simulink model "Saturation"  (R2022b)
settings: Solver=VariableStepAuto  StartTime=0.0  StopTime=10.0  RelTol=1e-3
settings Model: Creator=adlercohen  LastModifiedBy=adlercohen

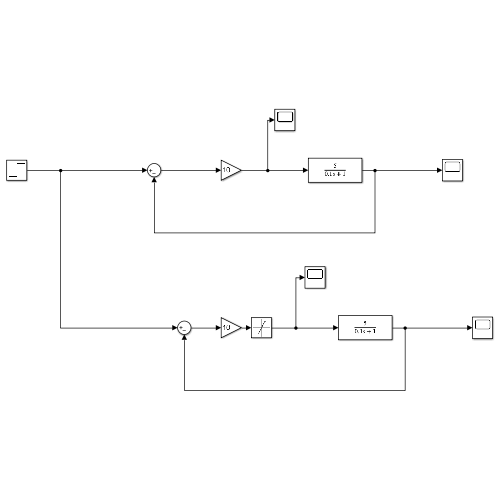
[thumbnail: Simulink's stored preview of the top-level diagram]
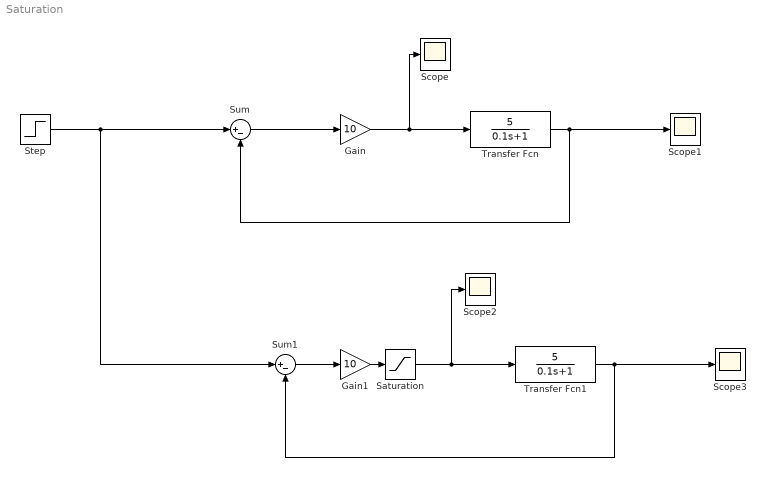
== system Saturation ==
  Gain : Gain  Gain=10
  Gain1 : Gain  Gain=10
  Saturation : Saturate  UpperLimit=5  LowerLimit=-5
  Scope{,1..3} (4 alike) : Scope
  Step : Step  Time=0  SampleTime=0
  Sum : Sum  Inputs=|+-
  Sum1 : Sum  Inputs=|+-
  Transfer Fcn : TransferFcn  Numerator=[5]  Denominator=[0.1 1]
  Transfer Fcn1 : TransferFcn  Numerator=[5]  Denominator=[0.1 1]
  wires:
  Gain/1 -> Scope/1, Transfer Fcn/1
  Sum/1 -> Gain/1
  Transfer Fcn/1 -> Scope1/1, Sum/2
  Sum1/1 -> Gain1/1
  Step/1 -> Sum1/1, Sum/1
  Transfer Fcn1/1 -> Scope3/1, Sum1/2
  Gain1/1 -> Saturation/1
  Saturation/1 -> Scope2/1, Transfer Fcn1/1
